simulink model "TA4sim"  (R2021a)
settings: Solver=VariableStepAuto  StartTime=0.0  StopTime=10.0  MaxStep=1e-4  RelTol=1e-3
values from neighbouring files (symbols this model uses):
  a0 = 30    [TA4.m]
  am1 = 2*zeta*wn    (= 7.8)    [TA4.m]    (also in WOZC.m = Am(2))
  am2 = wn^2    (= 36)    [TA4.m]    (also in WOZC.m = Am(3))
  P0 = 1e6*eye(3)    [TA4.m]
libraries: cstblocks x2
settings Model: Creator=ASUS  LastModifiedBy=ASUS

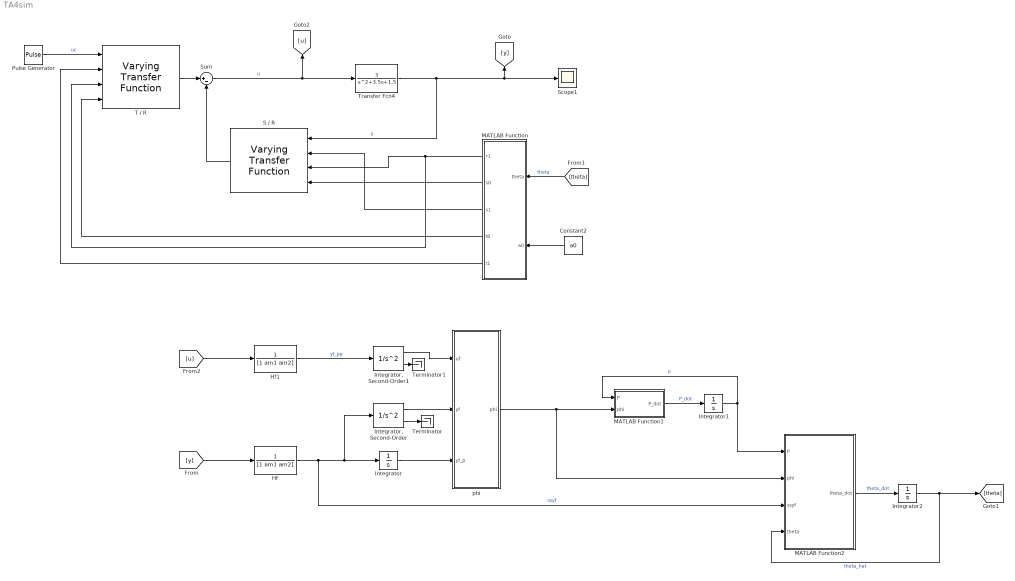
== system TA4sim ==
  Constant2 : Constant  Value=a0
  Hf : TransferFcn  Numerator=1  Denominator=[1 am1 am2]
  Hf1 : TransferFcn  Numerator=1  Denominator=[1 am1 am2]
  Integrator : Integrator
  "Integrator, Second-Order" : SecondOrderIntegrator
  "Integrator, Second-Order1" : SecondOrderIntegrator
  Integrator1 : Integrator  InitialCondition=P0
  Integrator2 : Integrator  InitialCondition=ones(3,1)
  MATLAB Function : MATLAB Function  TreatAsAtomicUnit=on
  MATLAB Function1 : MATLAB Function  TreatAsAtomicUnit=on
  MATLAB Function2 : MATLAB Function  TreatAsAtomicUnit=on
  Pulse Generator : DiscretePulseGenerator  PulseType=Time based  Period=5  PulseWidth=50
  S / R : cstblocks/Linear Parameter Varying/Varying Transfer Function  N=1
  Scope1 : Scope
  Sum : Sum  Inputs=|+-
  T / R : cstblocks/Linear Parameter Varying/Varying Transfer Function  N=1
  Terminator : Terminator
  Terminator1 : Terminator
  Transfer Fcn4 : TransferFcn  Numerator=[0 0 3]  Denominator=[1 3.5 1.5]
  phi : MATLAB Function  TreatAsAtomicUnit=on
  wires:
  Constant2/1 -> MATLAB Function/2(a0)
  [theta] -> MATLAB Function/1(theta)  "theta"
  MATLAB Function/1(r1) -> T / R/3, S / R/3
  MATLAB Function/2(s0) -> S / R/4
  MATLAB Function/3(s1) -> S / R/2
  Transfer Fcn4/1 -> [y], Scope1/1, S / R/1  "y"
  MATLAB Function/4(t0) -> T / R/4
  MATLAB Function/5(t1) -> T / R/2
  Pulse Generator/1 -> T / R/1  "uc"
  T / R/1 -> Sum/1
  S / R/1 -> Sum/2
  Sum/1 -> [u], Transfer Fcn4/1  "u"
  Hf/1 -> MATLAB Function2/3(ssyf), "Integrator, Second-Order"/1, Integrator/1  "ssyf"
  Hf1/1 -> "Integrator, Second-Order1"/1  "yf_pp"
  "Integrator, Second-Order"/1 -> phi/2(yf)
  Integrator/1 -> phi/3(yf_p)
  [y] -> Hf/1
  phi/1(phi) -> MATLAB Function2/2(phi), MATLAB Function1/2(phi)
  MATLAB Function1/1(P_dot) -> Integrator1/1  "P_dot"
  Integrator1/1 -> MATLAB Function2/1(P), MATLAB Function1/1(P)  "P"
  MATLAB Function2/1(theta_dot) -> Integrator2/1  "theta_dot"
  Integrator2/1 -> [theta], MATLAB Function2/4(theta)  "theta_hat"
  [u] -> Hf1/1
  "Integrator, Second-Order"/2 -> Terminator/1
  "Integrator, Second-Order1"/1 -> phi/1(uf)
  "Integrator, Second-Order1"/2 -> Terminator1/1

== matlab function TA4sim/phi ==
  data: uf input; yf input; yf_p input; phi output
function phi = fcn(uf, yf, yf_p)

phi = [-yf_p -yf uf]';

end

== matlab function TA4sim/MATLAB Function ==
  data: theta input; r1 output; a0 input; s0 output; s1 output; t0 output; t1 output
function [r1,s0,s1,t0,t1] = fcn(theta,a0)

wn = 6;
zeta = 0.65;

r1 = 2*zeta*wn + a0 -theta(1);
s0 = (wn^2 + 2*a0*zeta*wn - theta(1)*r1 - theta(2))/theta(3);
s1 = ((wn^2*a0)-theta(2)*r1)/theta(3);
t0 = wn^2/theta(3);
t1 = a0 * wn^2 /theta(3);

end

== matlab function TA4sim/MATLAB Function1 ==
  data: P input; P_dot output; phi input
function P_dot = fcn(P,phi)

alpha = 0.05;
P_dot = alpha * P - P * (phi * phi') * P;

end

== matlab function TA4sim/MATLAB Function2 ==
  data: P input; theta_dot output; phi input; ssyf input; theta input
function theta_dot = fcn(P, phi, ssyf, theta)

theta_dot = P*phi*(ssyf-phi'*theta);

end
